simulink model "PDQuadrotor2015a"  (R2017a)
settings: Solver=ode1  StartTime=0.0  StopTime=10.0  RelTol=1e-3  EnableMultiTasking=on
values from neighbouring files (symbols this model uses):
  b = 3.13*10^(-5)    (= 3.13e-05)    [Quadparameters.m]    (also in Quadparameters2.m)
  d = 7.5*10^(-7)    (= 7.5e-07)    [Quadparameters.m]    (also in Quadparameters2.m)
  g = 9.807    [Quadparameters.m]    (also in Quadparameters2.m = 9.81)
  Ix = 7.5*10^(-3)    (= 0.0075)    [Quadparameters.m]    (also in Quadparameters2.m)
  Iy = 7.5*10^(-3)    (= 0.0075)    [Quadparameters.m]    (also in Quadparameters2.m)
  Iz = 1.3*10^(-2)    (= 0.013)    [Quadparameters.m]    (also in Quadparameters2.m)
  Jr = 6.5*10^(-5)    (= 6.5e-05)    [Quadparameters.m]    (also in Quadparameters2.m)
  kdp = 8    [Quadparameters.m]    (also in Quadparameters2.m)
  kdps = 8.3996    [Quadparameters.m]    (also in Quadparameters2.m)
  kdt = 8.09    [Quadparameters.m]    (also in Quadparameters2.m)
  kdx = 4    [Quadparameters.m]    (also in Quadparameters2.m)
  kdy = 4    [Quadparameters.m]    (also in Quadparameters2.m)
  kdz = 13.795    [Quadparameters.m]    (also in Quadparameters2.m)
  kdz2 = 0.4    [Quadparameters.m]    (also in Quadparameters2.m)
  kpp = 50    [Quadparameters.m]    (also in Quadparameters2.m)
  kpps = 50    [Quadparameters.m]    (also in Quadparameters2.m)
  kpt = 50    [Quadparameters.m]    (also in Quadparameters2.m)
  kpx = 6    [Quadparameters.m]    (also in Quadparameters2.m)
  kpy = 6    [Quadparameters.m]    (also in Quadparameters2.m)
  kpz = 90    [Quadparameters.m]    (also in Quadparameters2.m)
  kpz2 = 6    [Quadparameters.m]    (also in Quadparameters2.m)
  l = 0.23    [Quadparameters.m]    (also in Quadparameters2.m)
  m = 0.65    [Quadparameters.m]    (also in Quadparameters2.m)
undefined symbols (not defined in the file or in its folder): magnitude
settings Model: Creator=abdelrazzak.merheb  LastModifiedBy=jean-marie
settings DataIOCC: LimitDataPoints=on  SaveFormat=Array  SignalLoggingSaveFormat=ModelDataLogs
settings OptimizationCC: ExpressionDepthLimit=2147483647
settings DebuggingCC: UnderspecifiedInitializationDetection=Classic  MergeDetectMultiDrivingBlocksExec=none  SolverPrmCheckMsg=warning  FcnCallInpInsideContextMsg=warning  StateNameClashWarn=warning  SFUnexpectedBacktrackingDiag=warning  SFNoUnconditionalDefaultTransitionDiag=warning  SFExecutionAtInitializationDiag=none
settings HardwareCC: ProdBitPerPointer=32  ProdBitPerSizeT=32  ProdBitPerPtrDiffT=32  ProdLargestAtomicFloat=None  ProdIntDivRoundTo=Undefined  ProdEndianess=Unspecified  ProdWordSize=32  ProdHWDeviceType=32-bit Generic
settings ModelReferenceCC: PropagateSignalLabelsOutOfModel=off
settings RTWCC: SystemTargetFile=fmu_cs2.tlc  MakeCommand=make_rtw FMIT_INTERMEDIATE_LIB_DIR=DEFAULT FMIT_ADDITIONAL_CFLAGS=  TemplateMakefile=fmu_cs2_default_tmf  Description=FMU Co-Simulation 2.0 Standalone  CheckMdlBeforeBuild=Warning
settings STFCustomTargetCC: ModelReferenceCompliant=off  MATLABClassNameForMDSCustomization=Simulink.SoftwareTarget.TargetSpecificTriggerConfigurationBase  SystemTargetFile=fmu_cs2.tlc
settings ConfigComp: CovMetricSettings=dw  CovHtmlReporting=on  CovSaveCumulativeToWorkspaceVar=on  CovSaveSingleToWorkspaceVar=on  CovExternalEMLEnable=off

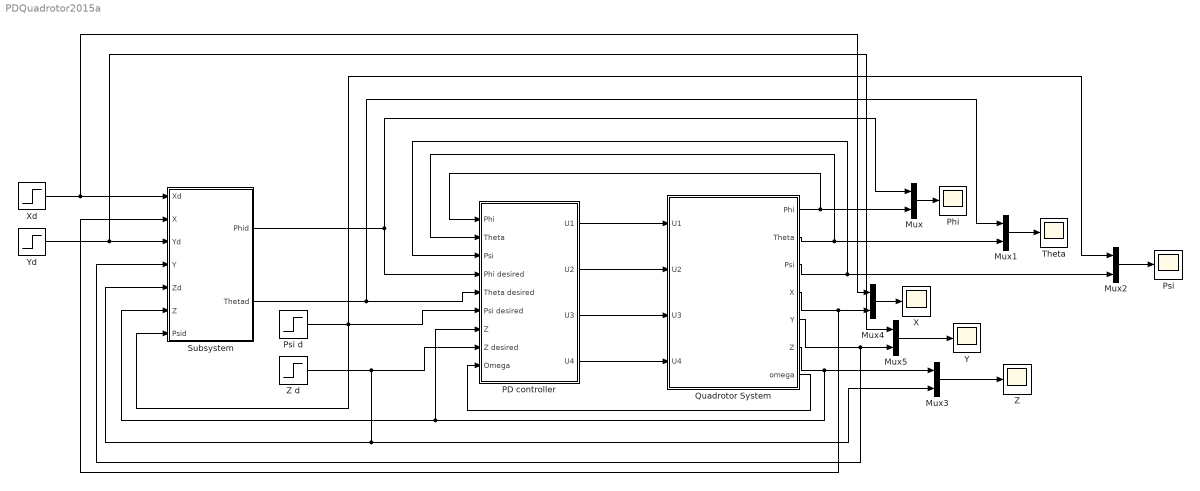
== system PDQuadrotor2015a ==
  Mux{,1..5} (6 alike) : Mux  Inputs=2
  PD controller : Subsystem
  Phi : Scope
  Psi : Scope
  Psi d : Step  SampleTime=0
  Quadrotor System : Subsystem
  Subsystem : Subsystem
  Theta : Scope
  X : Scope
  Xd : Step  After=5  SampleTime=0
  Y : Scope
  Yd : Step  After=5  SampleTime=0
  Z : Scope
  Z d : Step  SampleTime=0
  wires:
  PD controller/1(U1) -> Quadrotor System/1(U1)
  Quadrotor System/6(Z) -> Subsystem/6(Z), PD controller/7(Z), Mux3/1
  Quadrotor System/1(Phi) -> PD controller/1(Phi), Mux/2
  Quadrotor System/2(Theta) -> PD controller/2(Theta), Mux1/2
  Quadrotor System/3(Psi) -> PD controller/3(Psi), Mux2/2
  Subsystem/1(Phid) -> PD controller/4(Phi desired), Mux/1
  Subsystem/2(Thetad) -> Mux1/1, PD controller/5(Theta desired)
  Psi d/1 -> Subsystem/7(Psid), PD controller/6(Psi desired), Mux2/1
  Z d/1 -> PD controller/8(Z desired), Mux3/2, Subsystem/5(Zd)
  Quadrotor System/5(Y) -> Mux5/2, Subsystem/4(Y)
  Quadrotor System/4(X) -> Mux4/2, Subsystem/2(X)
  Mux/1 -> Phi/1
  Mux1/1 -> Theta/1
  Mux2/1 -> Psi/1
  Mux3/1 -> Z/1
  Xd/1 -> Mux4/1, Subsystem/1(Xd)
  Yd/1 -> Mux5/1, Subsystem/3(Yd)
  PD controller/2(U2) -> Quadrotor System/2(U2)
  PD controller/3(U3) -> Quadrotor System/3(U3)
  PD controller/4(U4) -> Quadrotor System/4(U4)
  Quadrotor System/7(omega) -> PD controller/9(Omega)
  Mux4/1 -> X/1
  Mux5/1 -> Y/1

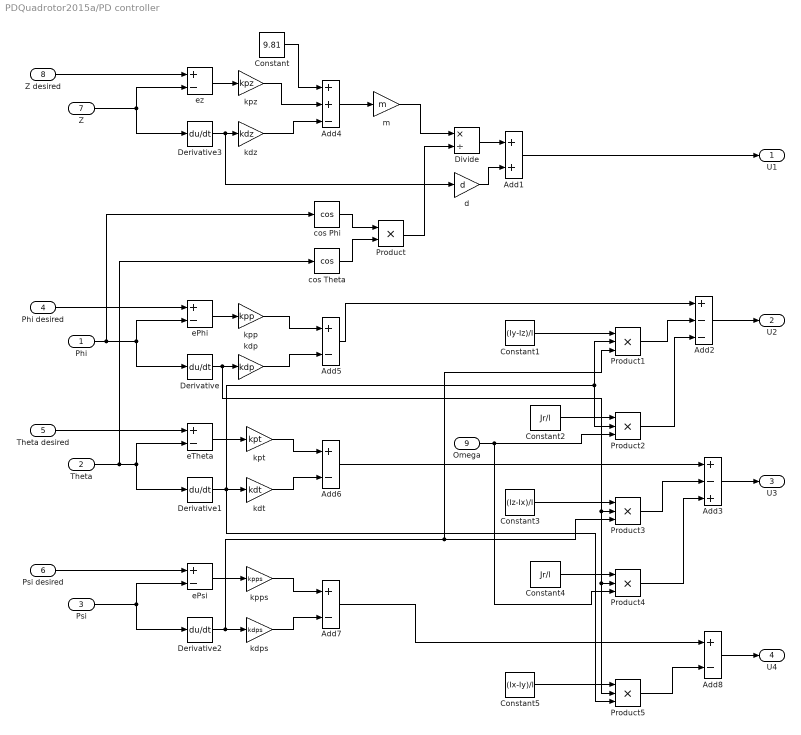
== system PDQuadrotor2015a/PD controller ==
  Phi : Inport
  Theta : Inport  Port=2
  Psi : Inport  Port=3
  Phi desired : Inport  Port=4
  Theta desired : Inport  Port=5
  Psi desired : Inport  Port=6
  Z : Inport  Port=7
  Z desired : Inport  Port=8
  Omega : Inport  Port=9
  Add1 : Sum
  Add2 : Sum  Inputs=+--
  Add3 : Sum  Inputs=+-+
  Add4 : Sum  Inputs=++-
  Add{5..8} (4 alike) : Sum  Inputs=+-
  Constant : Constant  Value=9.81
  Constant1 : Constant  Value=(Iy-Iz)/l
  Constant2 : Constant  Value=Jr/l
  Constant3 : Constant  Value=(Iz-Ix)/l
  Constant4 : Constant  Value=Jr/l
  Constant5 : Constant  Value=(Ix-Iy)/l
  Derivative{,1..3} (4 alike) : Derivative
  Divide : Product  Inputs=*/
  Product : Product  RndMeth=Zero
  Product{1..5} (5 alike) : Product  Inputs=3  RndMeth=Zero
  cos Phi : Trigonometry  Operator=cos
  cos Theta : Trigonometry  Operator=cos
  d : Gain  Gain=d
  ePhi : Sum  Inputs=+-
  ePsi : Sum  Inputs=+-
  eTheta : Sum  Inputs=+-
  ez : Sum  Inputs=+-
  kdp : Gain  Gain=kdp
  kdps : Gain  Gain=kdps
  kdt : Gain  Gain=kdt
  kdz : Gain  Gain=kdz
  kpp : Gain  Gain=kpp
  kpps : Gain  Gain=kpps
  kpt : Gain  Gain=kpt
  kpz : Gain  Gain=kpz
  m : Gain  Gain=m
  U1 : Outport
  U2 : Outport  Port=2
  U3 : Outport  Port=3
  U4 : Outport  Port=4
  wires:
  Phi/1 -> Derivative/1, ePhi/2, cos Phi/1
  Theta/1 -> Derivative1/1, eTheta/2, cos Theta/1
  Psi/1 -> Derivative2/1, ePsi/2
  Phi desired/1 -> ePhi/1
  Theta desired/1 -> eTheta/1
  Psi desired/1 -> ePsi/1
  ePhi/1 -> kpp/1
  eTheta/1 -> kpt/1
  ePsi/1 -> kpps/1
  Derivative2/1 -> Product3/3, Product1/3, kdps/1
  Z/1 -> Derivative3/1, ez/2
  Z desired/1 -> ez/1
  ez/1 -> kpz/1
  Derivative3/1 -> d/1, kdz/1
  kpp/1 -> Add5/1
  kdp/1 -> Add5/2
  Add5/1 -> Add2/1
  kpt/1 -> Add6/1
  kdt/1 -> Add6/2
  Add6/1 -> Add3/1
  kpps/1 -> Add7/1
  kdps/1 -> Add7/2
  Add7/1 -> Add8/1
  cos Phi/1 -> Product/1
  cos Theta/1 -> Product/2
  Add4/1 -> m/1
  m/1 -> Divide/1
  Product/1 -> Divide/2
  Constant/1 -> Add4/1
  kpz/1 -> Add4/2
  kdz/1 -> Add4/3
  Divide/1 -> Add1/1
  Add1/1 -> U1/1
  d/1 -> Add1/2
  Constant1/1 -> Product1/1
  Constant2/1 -> Product2/1
  Product1/1 -> Add2/2
  Product2/1 -> Add2/3
  Add2/1 -> U2/1
  Constant3/1 -> Product3/1
  Product3/1 -> Add3/2
  Derivative/1 -> Product3/2, Product4/2, Product5/2, kdp/1
  Constant4/1 -> Product4/1
  Omega/1 -> Product4/3, Product2/3
  Product4/1 -> Add3/3
  Add3/1 -> U3/1
  Derivative1/1 -> Product5/3, Product2/2, Product1/2, kdt/1
  Constant5/1 -> Product5/1
  Product5/1 -> Add8/2
  Add8/1 -> U4/1

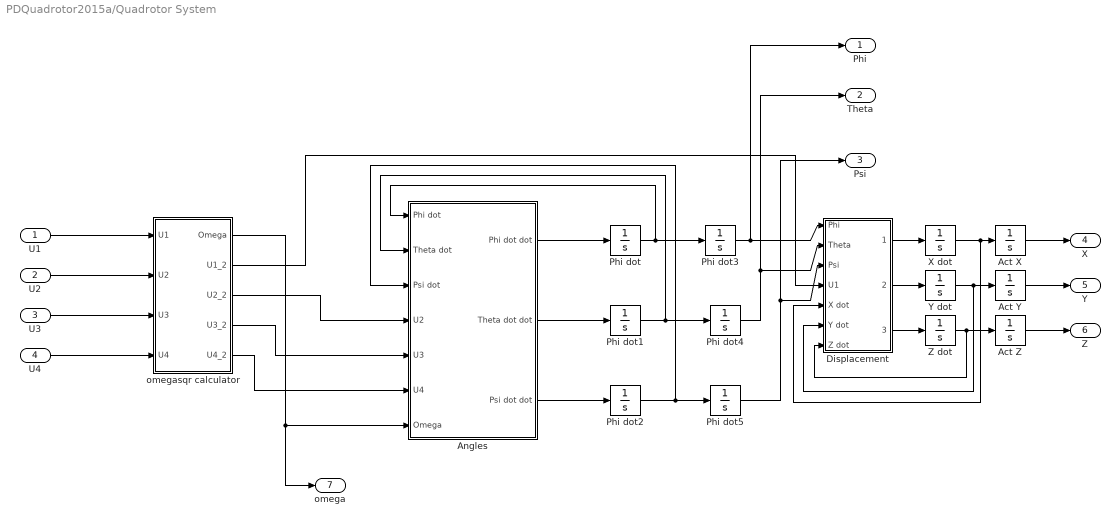
== system PDQuadrotor2015a/Quadrotor System ==
  U1 : Inport
  U2 : Inport  Port=2
  U3 : Inport  Port=3
  U4 : Inport  Port=4
  Act X : Integrator
  Act Y : Integrator
  Act Z : Integrator
  Angles : Subsystem
  Displacement : Subsystem
  Phi dot : Integrator
  Phi dot{1..5} (5 alike) : Integrator  ZeroCross=off
  X dot : Integrator
  Y dot : Integrator
  Z dot : Integrator
  omegasqr calculator : Subsystem
  Phi : Outport
  Theta : Outport  Port=2
  Psi : Outport  Port=3
  X : Outport  Port=4
  Y : Outport  Port=5
  Z : Outport  Port=6
  omega : Outport  Port=7
  wires:
  Angles/1(Phi dot dot) -> Phi dot/1
  Angles/2(Theta dot dot) -> Phi dot1/1
  Angles/3(Psi dot dot) -> Phi dot2/1
  Phi dot/1 -> Angles/1(Phi dot), Phi dot3/1
  Phi dot1/1 -> Angles/2(Theta dot), Phi dot4/1
  Phi dot2/1 -> Angles/3(Psi dot), Phi dot5/1
  omegasqr calculator/3(U2_2) -> Angles/4(U2)
  omegasqr calculator/4(U3_2) -> Angles/5(U3)
  omegasqr calculator/5(U4_2) -> Angles/6(U4)
  omegasqr calculator/1(Omega) -> omega/1, Angles/7(Omega)
  Phi dot3/1 -> Displacement/1(Phi), Phi/1
  Phi dot4/1 -> Displacement/2(Theta), Theta/1
  Phi dot5/1 -> Displacement/3(Psi), Psi/1
  omegasqr calculator/2(U1_2) -> Displacement/4(U1)
  X dot/1 -> Displacement/5(X dot), Act X/1
  Y dot/1 -> Displacement/6(Y dot), Act Y/1
  Displacement/1(x dotdot) -> X dot/1
  Z dot/1 -> Displacement/7(Z dot), Act Z/1
  Displacement/3(z dotdot) -> Z dot/1
  Act X/1 -> X/1
  Act Y/1 -> Y/1
  Act Z/1 -> Z/1
  U1/1 -> omegasqr calculator/1(U1)
  U2/1 -> omegasqr calculator/2(U2)
  U3/1 -> omegasqr calculator/3(U3)
  U4/1 -> omegasqr calculator/4(U4)
  Displacement/2(y dotdot) -> Y dot/1

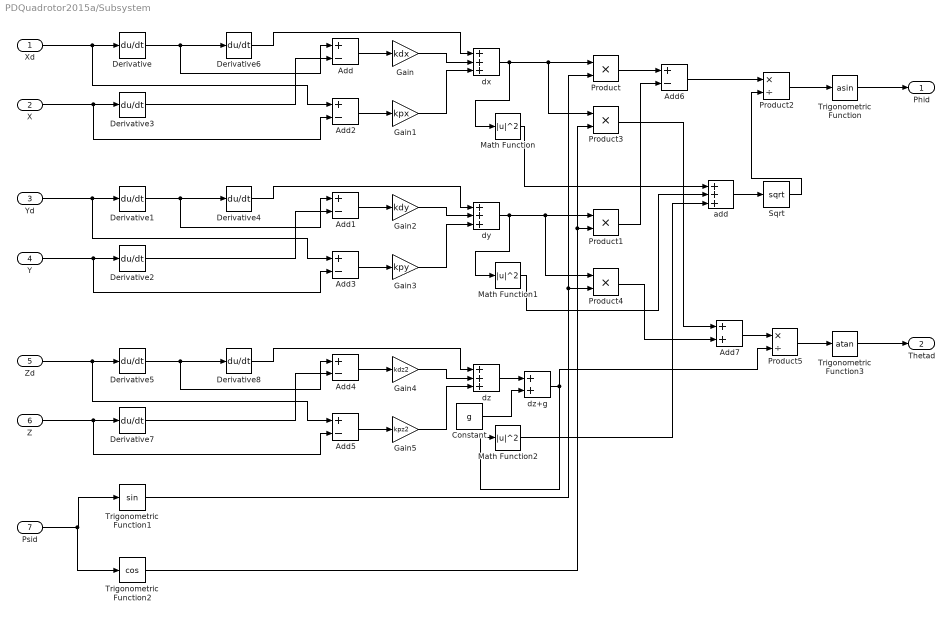
== system PDQuadrotor2015a/Subsystem ==
  Xd : Inport
  X : Inport  Port=2
  Yd : Inport  Port=3
  Y : Inport  Port=4
  Zd : Inport  Port=5
  Z : Inport  Port=6
  Psid : Inport  Port=7
  Add{,1..6} (7 alike) : Sum  Inputs=+-
  Add7 : Sum
  Constant : Constant  Value=g
  Derivative{,1..8} (9 alike) : Derivative
  Gain : Gain  Gain=kdx
  Gain1 : Gain  Gain=kpx
  Gain2 : Gain  Gain=kdy
  Gain3 : Gain  Gain=kpy
  Gain4 : Gain  Gain=kdz2
  Gain5 : Gain  Gain=kpz2
  Math Function : Math  Operator=magnitude^2  SaturateOnIntegerOverflow=on
  Math Function1 : Math  Operator=magnitude^2  SaturateOnIntegerOverflow=on
  Math Function2 : Math  Operator=magnitude^2  SaturateOnIntegerOverflow=on
  Product{,1,3..4} (4 alike) : Product
  Product2 : Product  Inputs=*/
  Product5 : Product  Inputs=*/
  Sqrt : Sqrt  SaturateOnIntegerOverflow=on
  Trigonometric Function : Trigonometry  Operator=asin
  Trigonometric Function1 : Trigonometry
  Trigonometric Function2 : Trigonometry  Operator=cos
  Trigonometric Function3 : Trigonometry  Operator=atan
  add : Sum  Inputs=+++
  dx : Sum  Inputs=+++
  dy : Sum  Inputs=+++
  dz : Sum  Inputs=+++
  dz+g : Sum
  Phid : Outport
  Thetad : Outport  Port=2
  wires:
  Sqrt/1 -> Product2/2
  Gain/1 -> dx/2
  Product3/1 -> Add7/1
  dz/1 -> dz+g/1
  Gain1/1 -> dx/3
  Constant/1 -> dz+g/2
  Xd/1 -> Add2/1, Derivative/1
  Derivative2/1 -> Add1/2
  X/1 -> Add2/2, Derivative3/1
  Derivative/1 -> Add/1, Derivative6/1
  Add/1 -> Gain/1
  Derivative3/1 -> Add/2
  Z/1 -> Add5/2, Derivative7/1
  Add3/1 -> Gain3/1
  Gain3/1 -> dy/3
  Derivative6/1 -> dx/1
  Add2/1 -> Gain1/1
  Derivative1/1 -> Add1/1, Derivative4/1
  Derivative8/1 -> dz/1
  Gain2/1 -> dy/2
  Derivative5/1 -> Add4/1, Derivative8/1
  Yd/1 -> Add3/1, Derivative1/1
  add/1 -> Sqrt/1
  Add6/1 -> Product2/1
  Derivative4/1 -> dy/1
  Y/1 -> Add3/2, Derivative2/1
  Product2/1 -> Trigonometric Function/1
  Add1/1 -> Gain2/1
  Math Function1/1 -> add/2
  Add5/1 -> Gain5/1
  Gain4/1 -> dz/2
  Zd/1 -> Add5/1, Derivative5/1
  Derivative7/1 -> Add4/2
  Gain5/1 -> dz/3
  Add4/1 -> Gain4/1
  Trigonometric Function1/1 -> Product4/2, Product/2
  Product1/1 -> Add6/2
  dx/1 -> Math Function/1, Product3/1, Product/1
  Math Function/1 -> add/1
  Product/1 -> Add6/1
  Trigonometric Function2/1 -> Product3/2, Product1/2
  Psid/1 -> Trigonometric Function2/1, Trigonometric Function1/1
  dy/1 -> Math Function1/1, Product4/1, Product1/1
  Math Function2/1 -> add/3
  Trigonometric Function3/1 -> Thetad/1
  Product4/1 -> Add7/2
  Product5/1 -> Trigonometric Function3/1
  Add7/1 -> Product5/1
  dz+g/1 -> Math Function2/1, Product5/2
  Trigonometric Function/1 -> Phid/1

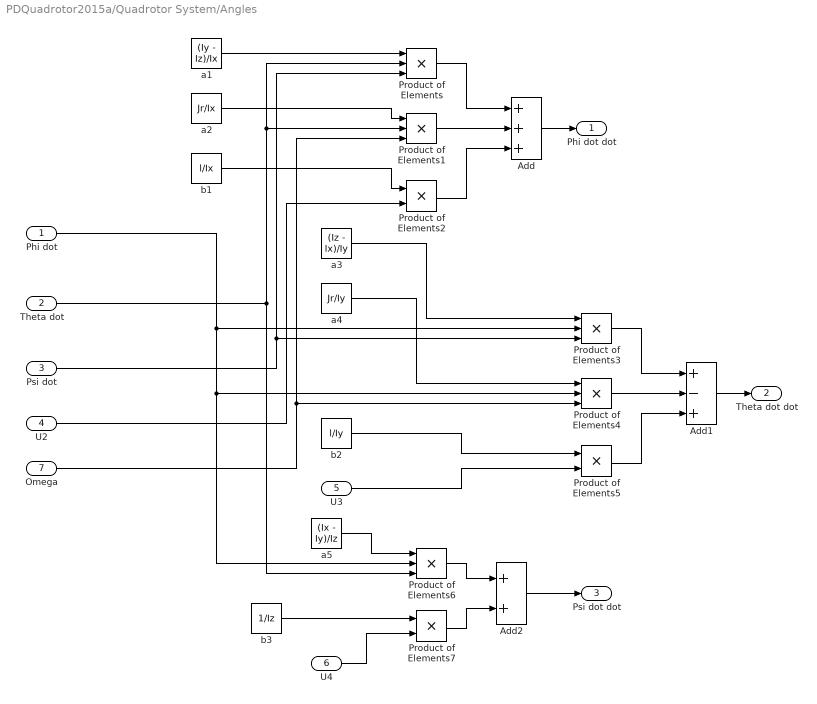
== system PDQuadrotor2015a/Quadrotor System/Angles ==
  Phi dot : Inport
  Theta dot : Inport  Port=2
  Psi dot : Inport  Port=3
  U2 : Inport  Port=4
  U3 : Inport  Port=5
  U4 : Inport  Port=6
  Omega : Inport  Port=7
  Add : Sum  Inputs=+++
  Add1 : Sum  Inputs=+-+
  Add2 : Sum
  Product of Elements{,1,3..4,6} (5 alike) : Product  Inputs=3
  Product of Elements2 : Product
  Product of Elements5 : Product
  Product of Elements7 : Product
  a1 : Constant  Value=(Iy - Iz)/Ix
  a2 : Constant  Value=Jr/Ix
  a3 : Constant  Value=(Iz - Ix)/Iy
  a4 : Constant  Value=Jr/Iy
  a5 : Constant  Value=(Ix - Iy)/Iz
  b1 : Constant  Value=l/Ix
  b2 : Constant  Value=l/Iy
  b3 : Constant  Value=1/Iz
  Phi dot dot : Outport
  Theta dot dot : Outport  Port=2
  Psi dot dot : Outport  Port=3
  wires:
  Product of Elements/1 -> Add/1
  Product of Elements1/1 -> Add/2
  Product of Elements2/1 -> Add/3
  Add/1 -> Phi dot dot/1
  a1/1 -> Product of Elements/1
  Theta dot/1 -> Product of Elements/2, Product of Elements1/2, Product of Elements6/3
  Psi dot/1 -> Product of Elements/3, Product of Elements3/3
  a2/1 -> Product of Elements1/1
  b1/1 -> Product of Elements2/1
  U2/1 -> Product of Elements2/2
  Omega/1 -> Product of Elements1/3, Product of Elements4/3
  Product of Elements3/1 -> Add1/1
  Product of Elements4/1 -> Add1/2
  Product of Elements5/1 -> Add1/3
  Add1/1 -> Theta dot dot/1
  a3/1 -> Product of Elements3/1
  a4/1 -> Product of Elements4/1
  b2/1 -> Product of Elements5/1
  U3/1 -> Product of Elements5/2
  Phi dot/1 -> Product of Elements3/2, Product of Elements4/2, Product of Elements6/2
  Product of Elements6/1 -> Add2/1
  Product of Elements7/1 -> Add2/2
  Add2/1 -> Psi dot dot/1
  U4/1 -> Product of Elements7/2
  b3/1 -> Product of Elements7/1
  a5/1 -> Product of Elements6/1

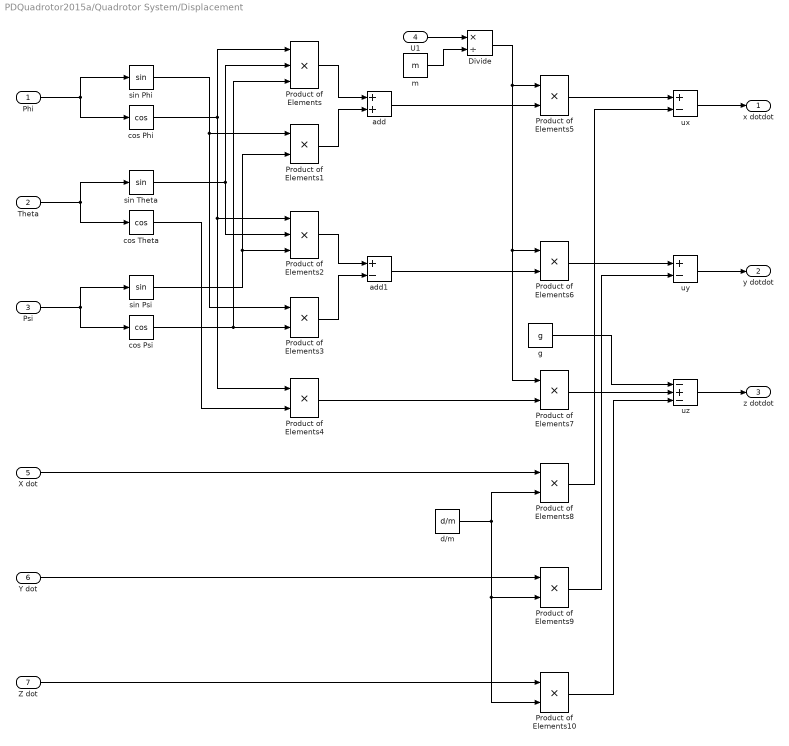
== system PDQuadrotor2015a/Quadrotor System/Displacement ==
  Phi : Inport
  Theta : Inport  Port=2
  Psi : Inport  Port=3
  U1 : Inport  Port=4
  X dot : Inport  Port=5
  Y dot : Inport  Port=6
  Z dot : Inport  Port=7
  Divide : Product  Inputs=*/
  Product of Elements : Product  Inputs=3
  Product of Elements{1,3..10} (9 alike) : Product
  Product of Elements2 : Product  Inputs=3
  add : Sum
  "add1 " : Sum  Inputs=+-
  cos Phi : Trigonometry  Operator=cos
  cos Psi : Trigonometry  Operator=cos
  cos Theta : Trigonometry  Operator=cos
  d/m : Constant  Value=d/m
  g : Constant  Value=g
  m : Constant  Value=m
  sin Phi : Trigonometry
  sin Psi : Trigonometry
  sin Theta : Trigonometry
  ux : Sum  Inputs=+-
  uy : Sum  Inputs=+-
  uz : Sum  Inputs=-+-
  x dotdot : Outport
  y dotdot : Outport  Port=2
  z dotdot : Outport  Port=3
  wires:
  Phi/1 -> sin Phi/1, cos Phi/1
  Theta/1 -> sin Theta/1, cos Theta/1
  Psi/1 -> sin Psi/1, cos Psi/1
  sin Theta/1 -> Product of Elements/2, Product of Elements2/2
  cos Psi/1 -> Product of Elements/3, Product of Elements3/2
  cos Phi/1 -> Product of Elements/1, Product of Elements2/1, Product of Elements4/1
  sin Phi/1 -> Product of Elements1/1, Product of Elements3/1
  sin Psi/1 -> Product of Elements1/2, Product of Elements2/3
  Product of Elements/1 -> add/1
  Product of Elements1/1 -> add/2
  add/1 -> Product of Elements5/2
  Product of Elements2/1 -> "add1 "/1
  Product of Elements3/1 -> "add1 "/2
  "add1 "/1 -> Product of Elements6/2
  cos Theta/1 -> Product of Elements4/2
  Product of Elements4/1 -> Product of Elements7/2
  U1/1 -> Divide/1
  m/1 -> Divide/2
  Divide/1 -> Product of Elements5/1, Product of Elements6/1, Product of Elements7/1
  Product of Elements5/1 -> ux/1
  Product of Elements6/1 -> uy/1
  uz/1 -> z dotdot/1
  Product of Elements7/1 -> uz/2
  g/1 -> uz/1
  X dot/1 -> Product of Elements8/1
  Y dot/1 -> Product of Elements9/1
  Z dot/1 -> Product of Elements10/1
  d/m/1 -> Product of Elements8/2, Product of Elements10/2, Product of Elements9/2
  Product of Elements10/1 -> uz/3
  Product of Elements8/1 -> ux/2
  Product of Elements9/1 -> uy/2
  ux/1 -> x dotdot/1
  uy/1 -> y dotdot/1

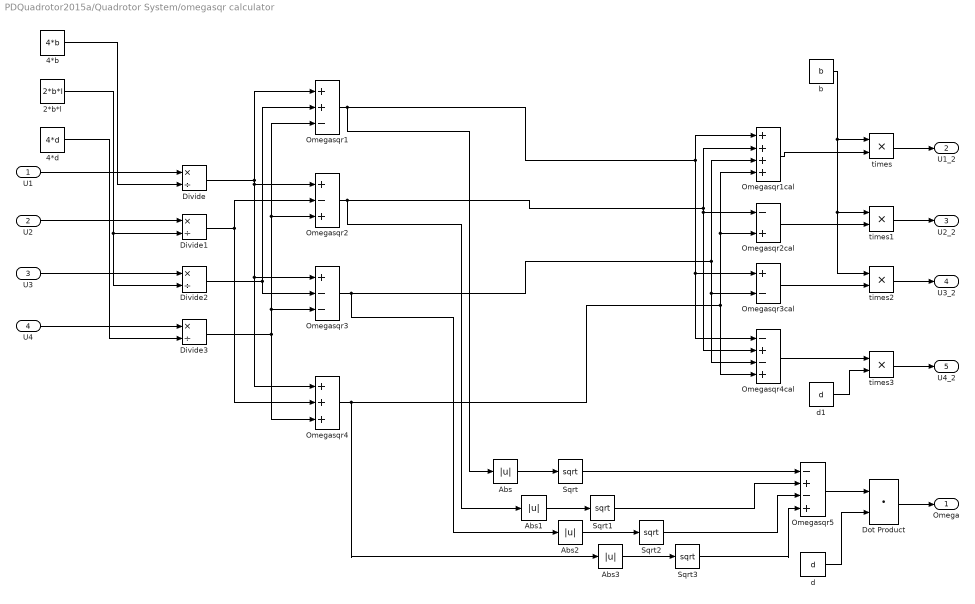
== system PDQuadrotor2015a/Quadrotor System/omegasqr calculator ==
  U1 : Inport
  U2 : Inport  Port=2
  U3 : Inport  Port=3
  U4 : Inport  Port=4
  2*b*l : Constant  Value=2*b*l
  4*b : Constant  Value=4*b
  4*d : Constant  Value=4*d
  Abs{,1..3} (4 alike) : Abs
  Divide{,1..3} (4 alike) : Product  Inputs=*/
  Dot Product : DotProduct  InputSameDT=on  OutDataTypeStr=Inherit: Inherit via internal rule
  Omegasqr1 : Sum  Inputs=++-
  Omegasqr1cal : Sum  Inputs=++++
  Omegasqr2 : Sum  Inputs=+-+
  Omegasqr2cal : Sum  Inputs=-+
  Omegasqr3 : Sum  Inputs=+--
  Omegasqr3cal : Sum  Inputs=+-
  Omegasqr4 : Sum  Inputs=+++
  Omegasqr4cal : Sum  Inputs=-+-+
  Omegasqr5 : Sum  Inputs=-+-+
  Sqrt{,1..3} (4 alike) : Sqrt  OutMin=[125]  OutMax=[523]  SaturateOnIntegerOverflow=on
  b : Constant  Value=b
  d : Constant  Value=d
  d1 : Constant  Value=d
  times{,1..3} (4 alike) : Product  Inputs=**
  Omega : Outport
  U1_2 : Outport  Port=2
  U2_2 : Outport  Port=3
  U3_2 : Outport  Port=4
  U4_2 : Outport  Port=5
  wires:
  U1/1 -> Divide/1
  4*b/1 -> Divide/2
  U2/1 -> Divide1/1
  2*b*l/1 -> Divide1/2, Divide2/2
  U3/1 -> Divide2/1
  U4/1 -> Divide3/1
  4*d/1 -> Divide3/2
  Divide/1 -> Omegasqr1/1, Omegasqr2/1, Omegasqr3/1, Omegasqr4/1
  Divide2/1 -> Omegasqr1/2, Omegasqr3/2
  Divide3/1 -> Omegasqr1/3, Omegasqr2/3, Omegasqr3/3, Omegasqr4/3
  Divide1/1 -> Omegasqr2/2, Omegasqr4/2
  Omegasqr1/1 -> Abs/1, Omegasqr1cal/1, Omegasqr3cal/1, Omegasqr4cal/1
  Omegasqr2/1 -> Abs1/1, Omegasqr1cal/2, Omegasqr2cal/1, Omegasqr4cal/2
  Omegasqr3/1 -> Abs2/1, Omegasqr1cal/3, Omegasqr3cal/2, Omegasqr4cal/3
  Omegasqr4/1 -> Abs3/1, Omegasqr1cal/4, Omegasqr2cal/2, Omegasqr4cal/4
  Omegasqr5/1 -> Dot Product/1
  Dot Product/1 -> Omega/1
  d/1 -> Dot Product/2
  b/1 -> times/1, times1/1, times2/1
  Omegasqr1cal/1 -> times/2
  Omegasqr2cal/1 -> times1/2
  Omegasqr3cal/1 -> times2/2
  Omegasqr4cal/1 -> times3/1
  d1/1 -> times3/2
  times/1 -> U1_2/1
  times1/1 -> U2_2/1
  times3/1 -> U4_2/1
  times2/1 -> U3_2/1
  Abs/1 -> Sqrt/1
  Abs1/1 -> Sqrt1/1
  Abs3/1 -> Sqrt3/1
  Abs2/1 -> Sqrt2/1
  Sqrt/1 -> Omegasqr5/1
  Sqrt1/1 -> Omegasqr5/2
  Sqrt2/1 -> Omegasqr5/3
  Sqrt3/1 -> Omegasqr5/4
